simulink model "Lab1PartA3"  (R2023a)
settings: Solver=VariableStepAuto  StartTime=0.0  StopTime=20.0  RelTol=1e-3
settings Model: Creator=m96sz  LastModifiedBy=m96sz

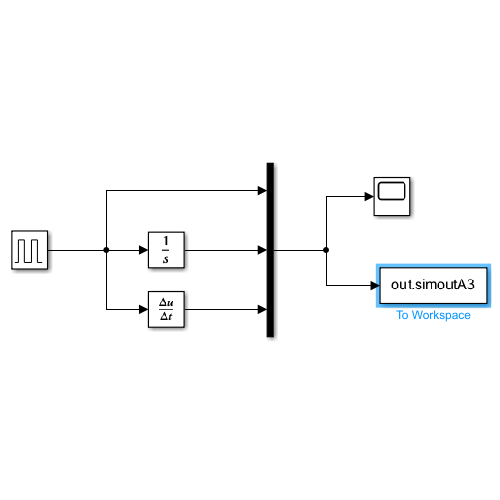
[thumbnail: Simulink's stored preview of the top-level diagram]
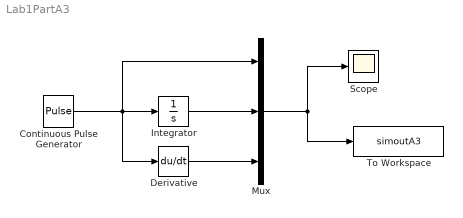
== system Lab1PartA3 ==
  Continuous Pulse Generator : DiscretePulseGenerator  PulseType=Time based  Period=5  PulseWidth=50
  Derivative : Derivative
  Integrator : Integrator
  Mux : Mux  Inputs=3
  Scope : Scope
  To Workspace : ToWorkspace  VariableName=simoutA3  SampleTime=-1
  wires:
  Integrator/1 -> Mux/2
  Continuous Pulse Generator/1 -> Mux/1, Derivative/1, Integrator/1
  Derivative/1 -> Mux/3
  Mux/1 -> Scope/1, To Workspace/1
